simulink model "RL_ML_System"  (R2019b)
settings: Solver=FixedStepAuto  StartTime=0.0  StopTime=10.0  RelTol=1e-3
values from neighbouring files (symbols this model uses):
  G = tf(num, den)    [controller_parameters_STUDENT.m]
  I0 = 0.69179046251    [controller.mat]    (also in controller_parameters_STUDENT.m = sqrt((2*g*m)/(Ld*cL))*(cL+Y0))
  U0 = 3.45895231255    [controller.mat]    (also in controller_parameters_STUDENT.m = R*I0)
  Y0 = 0.01    [controller.mat]    (also in controller_parameters_STUDENT.m)
settings Model: Creator=20201603  LastModifiedBy=s167385

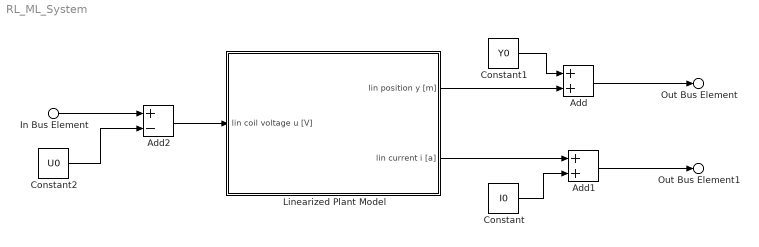
== system RL_ML_System ==
  In Bus Element : Inport  PortName=System_Control  Element=Voltage_PWM
  Add : Sum
  Add1 : Sum
  Add2 : Sum  Inputs=+-
  Constant : Constant  Value=I0
  Constant1 : Constant  Value=Y0
  Constant2 : Constant  Value=U0
  Linearized Plant Model : Subsystem
  Out Bus Element : Outport  PortName=Sensors  Element=Distance
  Out Bus Element1 : Outport  PortName=Sensors  Element=Current
  wires:
  Constant/1 -> Add1/2
  Add/1 -> Out Bus Element/1
  Linearized Plant Model/2(lin current i [a]) -> Add1/1
  Linearized Plant Model/1(lin position y [m]) -> Add/2
  Constant1/1 -> Add/1
  Add2/1 -> Linearized Plant Model/1(lin coil voltage u [V])
  In Bus Element/1 -> Add2/1
  Constant2/1 -> Add2/2
  Add1/1 -> Out Bus Element1/1

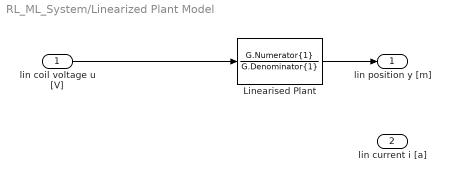
== system RL_ML_System/Linearized Plant Model ==
  lin coil voltage u [V] : Inport
  Linearised Plant : TransferFcn  Numerator=G.Numerator{1}  Denominator=G.Denominator{1}
  lin position y [m] : Outport
  lin current i [a] : Outport  Port=2
  wires:
  lin coil voltage u [V]/1 -> Linearised Plant/1
  Linearised Plant/1 -> lin position y [m]/1
